simulink model "M15"  (R2018a)
settings: Solver=VariableStepAuto  StartTime=0.0  StopTime=4  RelTol=1e-3
settings Model: Creator=admin  LastModifiedBy=admin

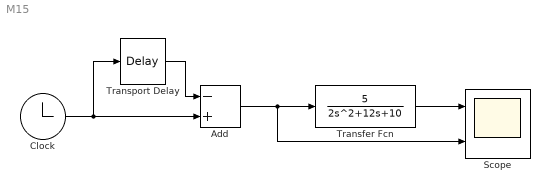
== system M15 ==
  Add : Sum  Inputs=-+
  Clock : Clock
  Scope : Scope  NumInputPorts=2
  Transfer Fcn : TransferFcn  Numerator=[5]  Denominator=[2 12 10]
  Transport Delay : TransportDelay  DelayTime=2
  wires:
  Clock/1 -> Transport Delay/1, Add/2
  Transport Delay/1 -> Add/1
  Add/1 -> Scope/2, Transfer Fcn/1
  Transfer Fcn/1 -> Scope/1
